simulink model "MPC_MEKF"  (R2024b)
settings: Solver=ode4  StartTime=0.0  StopTime=tsim  FixedStep=baseRate  RelTol=1e-6  AbsTol=1e-6
values from neighbouring files (symbols this model uses):
  D = zeros(3)    [MPC_Configuration.m]
  FOV = 120    [CV_Configuration.m]
  Gamma1_el = 0.12    [Run_Initializer.m]
  Gamma1_sh = 0.005    [Run_Initializer.m]
  Gamma1_wr = 0.025    [Run_Initializer.m]
  Gamma2_el = 5    [Run_Initializer.m]
  Gamma2_sh = 5    [Run_Initializer.m]
  Gamma2_wr = 5    [Run_Initializer.m]
  Gamma3_el = 10    [Run_Initializer.m]
  Gamma3_sh = 40    [Run_Initializer.m]
  Gamma3_wr = 40    [Run_Initializer.m]
  Gamma4_el = 0.039    [Run_Initializer.m]
  Gamma4_sh = 0.015    [Run_Initializer.m]
  Gamma4_wr = 0.029    [Run_Initializer.m]
  Gamma5_el = 800    [Run_Initializer.m]
  Gamma5_sh = 800    [Run_Initializer.m]
  Gamma5_wr = 800    [Run_Initializer.m]
  Gamma6_el = 0.000001    (= 1e-06)    [Run_Initializer.m]
  Gamma6_sh = 0.005    [Run_Initializer.m]
  Gamma6_wr = 0.02    [Run_Initializer.m]
  Kd_elarm = 0.8    [Run_Initializer.m]
  Kd_sharm = 1.0    (= 1)    [Run_Initializer.m]
  Kd_wrarm = 0.6    [Run_Initializer.m]
  kfObs = kfChaser    [PS_Filter_Config.m]
  kfTarget = kfChaser    [PS_Filter_Config.m]
  Kp_elarm = 1.2    [Run_Initializer.m]
  Kp_sharm = 1.5    [Run_Initializer.m]
  Kp_wrarm = 1.0    (= 1)    [Run_Initializer.m]
  M = 1    [MPC_Configuration.m]
  mpcIC = zeros((3*N + 6*N),1)    [MPC_Configuration.m]
  N = 15    [MPC_Configuration.m]    (also in PlotRawCV.m = length(time))
  PWMFreq = 5    [Run_Initializer.m]
  spotKFP0 = zeros(6,6,3)    [PS_Filter_Config.m]
  spotKFx0 = zeros(6,3)    [PS_Filter_Config.m]
  std = 1.5    [CV_Configuration.m]
  Tz_lim_elarm = .1    (= 0.1)    [Run_Initializer.m]
  Tz_lim_sharm = .1    (= 0.1)    [Run_Initializer.m]
  Tz_lim_wrarm = .1    (= 0.1)    [Run_Initializer.m]
  umax = T_max.*[1; 1; (0.3/2)]    [MPC_Configuration.m]
undefined symbols (not defined in the file or in its folder): a1, a2, a3, b0, b1, b2, b3, baseRate, dataRate, DiscIntNeverNeededParam, drop_states_ARM, drop_states_BLACK, drop_states_BLUE, drop_states_RED, F_black_X_nominal, F_black_Y_nominal, F_blue_X_nominal, F_blue_Y_nominal, F_red_X_nominal, F_red_Y_nominal, F_thrusters_BLACK, F_thrusters_BLUE, F_thrusters_RED, home_states_BLACK, home_states_BLUE, home_states_RED, IBLACK, IBLUE, IDIST, IEE, init_states_BLACK, init_states_BLUE, init_states_RED, IPROX, IRED, K_BLACK, K_BLUE, K_RED, Kd_tb, Kd_tblue, Kd_tr, Kd_xb, Kd_xblue, Kd_xr, Kd_yb, Kd_yblue, Kd_yr, kfChaser, Kp_tb, Kp_tblue, Kp_tr, Kp_xb, Kp_xblue, Kp_xr, Kp_yb, Kp_yblue, Kp_yr, mBLACK, mBLUE, mDIST ... (+23)
libraries: simulink x30, nvidiaSharedBlocks x13, MainLibrary x5, dspinverses x3, nvidiaIMUSensorslib x1
(part 2 of 8)

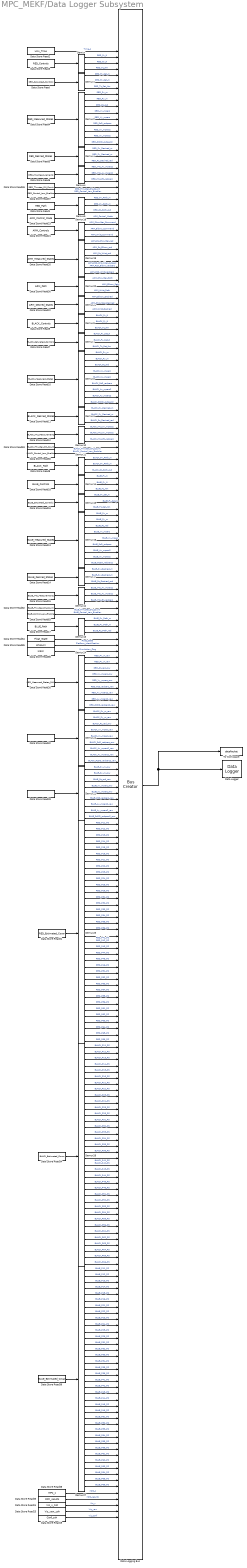
== system MPC_MEKF/Data Logger Subsystem ==
  Data Logger : MainLibrary/Data Logger  SystemSampleTime=-1  VariantActivationTime=update diagram  AllowFlexibleInterface=on  Latency=0  AutoFrameSizeCalculation=off
      settings: SourceProductName=SPOT Custom Library
  Data Logging Bus : BusCreator  Inputs=238
  Data Store Read : DataStoreRead  DataStoreName=RED_Saturated_Controls  IndexOptions=Index vector (dialog)  Indices=1  OutputSizes=1
  Data Store Read1 : DataStoreRead  DataStoreName=RED_Path  IndexOptions=Index vector (dialog)  Indices=1  OutputSizes=1
  Data Store Read10 : DataStoreRead  DataStoreName=BLACK_Measured_States  IndexOptions=Index vector (dialog)  Indices=1  OutputSizes=1
  Data Store Read11 : DataStoreRead  DataStoreName=BLACK_Desired_States  IndexOptions=Index vector (dialog)  Indices=1  OutputSizes=1
  Data Store Read12 : DataStoreRead  DataStoreName=BLACK_IMU_Measurements  IndexOptions=Index vector (dialog)  Indices=1  OutputSizes=1
  Data Store Read13 : DataStoreRead  DataStoreName=BLUE_Measured_States  IndexOptions=Index vector (dialog)  Indices=1  OutputSizes=1
  Data Store Read14 : DataStoreRead  DataStoreName=BLUE_Desired_States  IndexOptions=Index vector (dialog)  Indices=1  OutputSizes=1
  Data Store Read15 : DataStoreRead  DataStoreName=BLUE_IMU_Measurements  IndexOptions=Index vector (dialog)  Indices=1  OutputSizes=1
  Data Store Read16 : DataStoreRead  DataStoreName=BLUE_Saturated_Controls  IndexOptions=Index vector (dialog)  Indices=1  OutputSizes=1
  Data Store Read17 : DataStoreRead  DataStoreName=BLUE_Path  IndexOptions=Index vector (dialog)  Indices=1  OutputSizes=1
  Data Store Read18 : DataStoreRead  DataStoreName=BLUE_Controls  IndexOptions=Index vector (dialog)  Indices=1  OutputSizes=1
  Data Store Read19 : DataStoreRead  DataStoreName=Conf_zoh  IndexOptions=Index vector (dialog)  Indices=1  OutputSizes=1
  Data Store Read2 : DataStoreRead  DataStoreName=Univ_Time  IndexOptions=Index vector (dialog)  Indices=1  OutputSizes=1
  Data Store Read20 : DataStoreRead  DataStoreName=ARM_Measured_States  IndexOptions=Index vector (dialog)  Indices=1  OutputSizes=1
  Data Store Read21 : DataStoreRead  DataStoreName=ARM_Controls  IndexOptions=Index vector (dialog)  Indices=1  OutputSizes=1
  Data Store Read22 : DataStoreRead  DataStoreName=ARM_Desired_States  IndexOptions=Index vector (dialog)  Indices=1  OutputSizes=1
  Data Store Read23 : DataStoreRead  DataStoreName=ARM_Control_Mode  IndexOptions=Index vector (dialog)  Indices=1  OutputSizes=1
  Data Store Read24 : DataStoreRead  DataStoreName=Vis_x_zoh  IndexOptions=Index vector (dialog)  Indices=1  OutputSizes=1
  Data Store Read25 : DataStoreRead  DataStoreName=Vis_yaw_zoh  IndexOptions=Index vector (dialog)  Indices=1  OutputSizes=1
  Data Store Read26 : DataStoreRead  DataStoreName=RED_Measured_States_RAW  IndexOptions=Index vector (dialog)  Indices=1  OutputSizes=1
  Data Store Read28 : DataStoreRead  DataStoreName=BLUE_Measured_States_RAW  IndexOptions=Index vector (dialog)  Indices=1  OutputSizes=1
  Data Store Read3 : DataStoreRead  DataStoreName=RED_Controls  IndexOptions=Index vector (dialog)  Indices=1  OutputSizes=1
  Data Store Read30 : DataStoreRead  DataStoreName=ARM_Path  IndexOptions=Index vector (dialog)  Indices=1  OutputSizes=1
  Data Store Read31 : DataStoreRead  DataStoreName=RED_Estimated_Covar  IndexOptions=Index vector (dialog)  Indices=1  OutputSizes=1
  Data Store Read32 : DataStoreRead  DataStoreName=BLACK_Measured_States_RAW  IndexOptions=Index vector (dialog)  Indices=1  OutputSizes=1
  Data Store Read34 : DataStoreRead  DataStoreName=BLACK_Estimated_Covar  IndexOptions=Index vector (dialog)  Indices=1  OutputSizes=1
  Data Store Read35 : DataStoreRead  DataStoreName=MPC_results  IndexOptions=Index vector (dialog)  Indices=1  OutputSizes=1
  Data Store Read36 : DataStoreRead  DataStoreName=RED_Thruster_ON_Count  IndexOptions=Index vector (dialog)  Indices=1  OutputSizes=1
  Data Store Read37 : DataStoreRead  DataStoreName=RED_Control_Law_Enabler  IndexOptions=Index vector (dialog)  Indices=1  OutputSizes=1
  Data Store Read38 : DataStoreRead  DataStoreName=MPC_z  IndexOptions=Index vector (dialog)  Indices=1  OutputSizes=1
  Data Store Read39 : DataStoreRead  DataStoreName=BLUE_Estimated_Covar  IndexOptions=Index vector (dialog)  Indices=1  OutputSizes=1
  Data Store Read4 : DataStoreRead  DataStoreName=RED_Measured_States  IndexOptions=Index vector (dialog)  Indices=1  OutputSizes=1
  Data Store Read5 : DataStoreRead  DataStoreName=RED_Desired_States  IndexOptions=Index vector (dialog)  Indices=1  OutputSizes=1
  Data Store Read59 : DataStoreRead  DataStoreName=BLACK_Thruster_ON_Count  IndexOptions=Index vector (dialog)  Indices=1  OutputSizes=1
  Data Store Read6 : DataStoreRead  DataStoreName=RED_IMU_Measurements  IndexOptions=Index vector (dialog)  Indices=1  OutputSizes=1
  Data Store Read60 : DataStoreRead  DataStoreName=BLACK_Control_Law_Enabler  IndexOptions=Index vector (dialog)  Indices=1  OutputSizes=1
  Data Store Read7 : DataStoreRead  DataStoreName=BLACK_Saturated_Controls  IndexOptions=Index vector (dialog)  Indices=1  OutputSizes=1
  Data Store Read8 : DataStoreRead  DataStoreName=BLACK_Path  IndexOptions=Index vector (dialog)  Indices=1  OutputSizes=1
  Data Store Read82 : DataStoreRead  DataStoreName=BLUE_Thruster_ON_Count  IndexOptions=Index vector (dialog)  Indices=1  OutputSizes=1
  Data Store Read83 : DataStoreRead  DataStoreName=BLUE_Control_Law_Enabler  IndexOptions=Index vector (dialog)  Indices=1  OutputSizes=1
  Data Store Read84 : DataStoreRead  DataStoreName=Float_State  IndexOptions=Index vector (dialog)  Indices=1  OutputSizes=1
  Data Store Read85 : DataStoreRead  DataStoreName=WhoAmI  IndexOptions=Index vector (dialog)  Indices=1  OutputSizes=1
  Data Store Read86 : DataStoreRead  DataStoreName=isSim  IndexOptions=Index vector (dialog)  Indices=1  OutputSizes=1
  Data Store Read9 : DataStoreRead  DataStoreName=BLACK_Controls  IndexOptions=Index vector (dialog)  Indices=1  OutputSizes=1
  Demux{,1,3..7,9..15,17..18,20..21} (18 alike) : Demux  Outputs=3
  Demux{2,8,16,22..24} (6 alike) : Demux  Outputs=9
  Demux19 : Demux  Outputs=6
  Demux25 : Demux  Outputs=36
  Demux26 : Demux  Outputs=36
  Demux27 : Demux  Outputs=36
  To Workspace : ToWorkspace  VariableName=dataPacket  SaveFormat=Timeseries  SampleTime=-1
      settings: Save2DSignal=2-D array (concatenate along first dimension)
  wires:
  Data Logging Bus/1 -> To Workspace/1, Data Logger/1
  Demux6/1 -> Data Logging Bus/44  "BLACK_Fx_N"
  Demux6/2 -> Data Logging Bus/45  "BLACK_Fy_N"
  Demux6/3 -> Data Logging Bus/46  "BLACK_Tz_Nm"
  Demux7/1 -> Data Logging Bus/47  "BLACK_Fx_Sat_N"
  Demux7/2 -> Data Logging Bus/48  "BLACK_Fy_Sat_N"
  Demux7/3 -> Data Logging Bus/49  "BLACK_Tz_Sat_Nm"
  Demux8/1 -> Data Logging Bus/50  "BLACK_Px_m"
  Demux8/2 -> Data Logging Bus/51  "BLACK_Py_m"
  Demux8/3 -> Data Logging Bus/52  "BLACK_Rz_rad"
  Demux8/4 -> Data Logging Bus/53  "BLACK_Vx_mpers"
  Demux8/5 -> Data Logging Bus/54  "BLACK_Vy_mpers"
  Demux8/6 -> Data Logging Bus/55  "BLACK_RzD_radpers"
  Demux8/7 -> Data Logging Bus/56  "BLACK_Ax_mpers2"
  Demux8/8 -> Data Logging Bus/57  "BLACK_Ay_mpers2"
  Demux8/9 -> Data Logging Bus/58  "BLACK_RzDD_radpers2"
  Demux9/1 -> Data Logging Bus/59  "BLACK_Px_Desired_m"
  Demux9/2 -> Data Logging Bus/60  "BLACK_Py_Desired_m"
  Demux9/3 -> Data Logging Bus/61  "BLACK_Rz_Desired_rad"
  Demux10/1 -> Data Logging Bus/62  "BLACK_IMU_Ax_mpers2"
  Demux10/2 -> Data Logging Bus/63  "BLACK_IMU_Ay_mpers2"
  Demux10/3 -> Data Logging Bus/64  "BLACK_IMU_Gz_radpers"
  Demux11/1 -> Data Logging Bus/67  "BLACK_Px_Path_m"
  Demux11/2 -> Data Logging Bus/68  "BLACK_Py_Path_m"
  Demux11/3 -> Data Logging Bus/69  "BLACK_Rz_Path_rad"
  Demux14/1 -> Data Logging Bus/70  "BLUE_Fx_N"
  Demux14/2 -> Data Logging Bus/71  "BLUE_Fy_N"
  Demux14/3 -> Data Logging Bus/72  "BLUE_Tz_Nm"
  Demux15/1 -> Data Logging Bus/73  "BLUE_Fx_Sat_N"
  Demux15/2 -> Data Logging Bus/74  "BLUE_Fy_Sat_N"
  Demux15/3 -> Data Logging Bus/75  "BLUE_Tz_Sat_Nm"
  Demux16/1 -> Data Logging Bus/76  "BLUE_Px_m"
  Demux16/2 -> Data Logging Bus/77  "BLUE_Py_m"
  Demux16/3 -> Data Logging Bus/78  "BLUE_Rz_rad"
  Demux16/4 -> Data Logging Bus/79  "BLUE_Vx_mpers"
  Demux16/5 -> Data Logging Bus/80  "BLUE_Vy_mpers"
  Demux16/6 -> Data Logging Bus/81  "BLUE_RzD_radpers"
  Demux16/7 -> Data Logging Bus/82  "BLUE_Ax_mpers2"
  Demux16/8 -> Data Logging Bus/83  "BLUE_Ay_mpers2"
  Demux16/9 -> Data Logging Bus/84  "BLUE_RzDD_radpers2"
  Demux17/1 -> Data Logging Bus/85  "BLUE_Px_Desired_m"
  Demux17/2 -> Data Logging Bus/86  "BLUE_Py_Desired_m"
  Demux17/3 -> Data Logging Bus/87  "BLUE_Rz_Desired_rad"
  Demux12/1 -> Data Logging Bus/88  "BLUE_IMU_Ax_mpers2"
  Demux12/2 -> Data Logging Bus/89  "BLUE_IMU_Ay_mpers2"
  Demux12/3 -> Data Logging Bus/90  "BLUE_IMU_Gz_radpers"
  Data Store Read82/1 -> Data Logging Bus/91  "BLUE_Thruster_ON_Count"
  Data Store Read83/1 -> Data Logging Bus/92  "BLUE_Control_Law_Enabler"
  Demux13/1 -> Data Logging Bus/93  "BLUE_Px_Path_m"
  Demux13/2 -> Data Logging Bus/94  "BLUE_Py_Path_m"
  Demux13/3 -> Data Logging Bus/95  "BLUE_Rz_Path_rad"
  Data Store Read86/1 -> Data Logging Bus/98  "Simulation_Flag"
  Demux21/3 -> Data Logging Bus/43  "ARM_Wrist_Desired"
  Demux21/2 -> Data Logging Bus/42  "ARM_Shoulder_Desired"
  Demux21/1 -> Data Logging Bus/41  "ARM_Elbow_Desired"
  Demux20/3 -> Data Logging Bus/40  "ARM_Wrist_Path"
  Demux20/2 -> Data Logging Bus/39  "ARM_Elbow_Path"
  Data Store Read23/1 -> Data Logging Bus/28  "ARM_Control_Mode"
  Demux18/1 -> Data Logging Bus/29  "ARM_Shoulder_Command"
  Demux18/2 -> Data Logging Bus/30  "ARM_Elbow_Command"
  Demux18/3 -> Data Logging Bus/31  "ARM_Wrist_Command"
  Demux19/1 -> Data Logging Bus/32  "ARM_Rz_Shoulder_rad"
  Demux19/2 -> Data Logging Bus/33  "ARM_Rz_Elbow_rad"
  Demux19/3 -> Data Logging Bus/34  "ARM_Rz_Wrist_rad"
  Demux19/4 -> Data Logging Bus/35  "ARM_RzD_Shoulder_radpers"
  Demux19/5 -> Data Logging Bus/36  "ARM_RzD_Elbow_radpers"
  Demux19/6 -> Data Logging Bus/37  "ARM_RzD_Wrist_radpers"
  Demux20/1 -> Data Logging Bus/38  "ARM_Shoulder_Path"
  Data Store Read2/1 -> Data Logging Bus/1  "Time_s"
  Demux/1 -> Data Logging Bus/2  "RED_Fx_N"
  Demux/2 -> Data Logging Bus/3  "RED_Fy_N"
  Demux/3 -> Data Logging Bus/4  "RED_Tz_Nm"
  Demux1/1 -> Data Logging Bus/5  "RED_Fx_Sat_N"
  Demux1/2 -> Data Logging Bus/6  "RED_Fy_Sat_N"
  Demux1/3 -> Data Logging Bus/7  "RED_Tz_Sat_Nm"
  Demux2/1 -> Data Logging Bus/8  "RED_Px_m"
  Demux2/2 -> Data Logging Bus/9  "RED_Py_m"
  Demux2/3 -> Data Logging Bus/10  "RED_Rz_rad"
  Demux2/4 -> Data Logging Bus/11  "RED_Vx_mpers"
  Demux2/5 -> Data Logging Bus/12  "RED_Vy_mpers"
  Demux2/6 -> Data Logging Bus/13  "RED_RzD_radpers"
  Demux2/7 -> Data Logging Bus/14  "RED_Ax_mpers2"
  Demux2/8 -> Data Logging Bus/15  "RED_Ay_mpers2"
  Demux2/9 -> Data Logging Bus/16  "RED_RzDD_radpers2"
  Demux3/1 -> Data Logging Bus/17  "RED_Px_Desired_m"
  Demux3/2 -> Data Logging Bus/18  "RED_Py_Desired_m"
  Demux3/3 -> Data Logging Bus/19  "RED_Rz_Desired_rad"
  Demux4/1 -> Data Logging Bus/20  "RED_IMU_Ax_mpers2"
  Demux4/2 -> Data Logging Bus/21  "RED_IMU_Ay_mpers2"
  Demux4/3 -> Data Logging Bus/22  "RED_IMU_Gz_radpers"
  Data Store Read36/1 -> Data Logging Bus/23  "RED_Thruster_ON_Count"
  Data Store Read37/1 -> Data Logging Bus/24  "RED_Control_Law_Enabler"
  Demux5/1 -> Data Logging Bus/25  "RED_Px_Path_m"
  Demux5/2 -> Data Logging Bus/26  "RED_Py_Path_m"
  Demux5/3 -> Data Logging Bus/27  "RED_Rz_Path_rad"
  Data Store Read/1 -> Demux1/1
  Data Store Read3/1 -> Demux/1
  Data Store Read4/1 -> Demux2/1
  Data Store Read5/1 -> Demux3/1
  Data Store Read6/1 -> Demux4/1
  Data Store Read1/1 -> Demux5/1
  Data Store Read12/1 -> Demux10/1
  Data Store Read8/1 -> Demux11/1
  Data Store Read10/1 -> Demux8/1
  Data Store Read7/1 -> Demux7/1
  Data Store Read9/1 -> Demux6/1
  Data Store Read11/1 -> Demux9/1
  Data Store Read18/1 -> Demux14/1
  Data Store Read17/1 -> Demux13/1
  Data Store Read13/1 -> Demux16/1
  Data Store Read16/1 -> Demux15/1
  Data Store Read15/1 -> Demux12/1
  Data Store Read14/1 -> Demux17/1
  Data Store Read21/1 -> Demux18/1
  Data Store Read20/1 -> Demux19/1
  Data Store Read30/1 -> Demux20/1
  Data Store Read22/1 -> Demux21/1
  Data Store Read85/1 -> Data Logging Bus/97  "Platform_Identification"
  Data Store Read59/1 -> Data Logging Bus/65  "BLACK_Thruster_ON_Count"
  Data Store Read60/1 -> Data Logging Bus/66  "BLACK_Control_Law_Enabler"
  Data Store Read84/1 -> Data Logging Bus/96  "Float_State"
  Demux24/1 -> Data Logging Bus/99  "RED_Px_m_raw"
  Demux22/9 -> Data Logging Bus/125  "BLUE_RzDD_radpers2_raw"
  Data Store Read26/1 -> Demux24/1
  Demux24/2 -> Data Logging Bus/100  "RED_Py_m_raw"
  Demux24/3 -> Data Logging Bus/101  "RED_Rz_rad_raw"
  Demux24/4 -> Data Logging Bus/102  "RED_Vx_mpers_raw"
  Demux24/5 -> Data Logging Bus/103  "RED_Vy_mpers_raw"
  Demux24/6 -> Data Logging Bus/104  "RED_RzD_radpers_raw"
  Demux24/7 -> Data Logging Bus/105  "RED_Ax_mpers2_raw"
  Demux24/8 -> Data Logging Bus/106  "RED_Ay_mpers2_raw"
  Demux24/9 -> Data Logging Bus/107  "RED_RzDD_radpers2_raw"
  Demux23/1 -> Data Logging Bus/108  "BLACK_Px_m_raw"
  Demux23/2 -> Data Logging Bus/109  "BLACK_Py_m_raw"
  Demux23/3 -> Data Logging Bus/110  "BLACK_Rz_rad_raw"
  Demux23/4 -> Data Logging Bus/111  "BLACK_Vx_mpers_raw"
  Demux23/5 -> Data Logging Bus/112  "BLACK_Vy_mpers_raw"
  Demux23/6 -> Data Logging Bus/113  "BLACK_RzD_radpers_raw"
  Demux23/7 -> Data Logging Bus/114  "BLACK_Ax_mpers2_raw"
  Demux23/8 -> Data Logging Bus/115  "BLACK_Ay_mpers2_raw"
  Demux23/9 -> Data Logging Bus/116  "BLACK_RzDD_radpers2_raw"
  Data Store Read32/1 -> Demux23/1
  Demux22/1 -> Data Logging Bus/117  "BLUE_Px_m_raw"
  Demux22/2 -> Data Logging Bus/118  "BLUE_Py_m_raw"
  Demux22/3 -> Data Logging Bus/119  "BLUE_Rz_rad_raw"
  Demux22/4 -> Data Logging Bus/120  "BLUE_Vx_mpers_raw"
  Demux22/5 -> Data Logging Bus/121  "BLUE_Vy_mpers_raw"
  Demux22/6 -> Data Logging Bus/122  "BLUE_RzD_radpers_raw"
  Demux22/7 -> Data Logging Bus/123  "BLUE_Ax_mpers2_raw"
  Demux22/8 -> Data Logging Bus/124  "BLUE_Ay_mpers2_raw"
  Data Store Read28/1 -> Demux22/1
  Demux25/1 -> Data Logging Bus/126  "RED_P11_PS"
  Demux25/2 -> Data Logging Bus/127  "RED_P12_PS"
  Demux25/3 -> Data Logging Bus/128  "RED_P13_PS"
  Demux25/4 -> Data Logging Bus/129  "RED_P14_PS"
  Demux25/5 -> Data Logging Bus/130  "RED_P15_PS"
  Demux25/6 -> Data Logging Bus/131  "RED_P16_PS"
  Demux25/7 -> Data Logging Bus/132  "RED_P21_PS"
  Demux25/8 -> Data Logging Bus/133  "RED_P22_PS"
  Demux25/9 -> Data Logging Bus/134  "RED_P23_PS"
  Demux25/10 -> Data Logging Bus/135  "RED_P24_PS"
  Demux25/11 -> Data Logging Bus/136  "RED_P25_PS"
  Demux25/12 -> Data Logging Bus/137  "RED_P26_PS"
  Demux25/13 -> Data Logging Bus/138  "RED_P31_PS"
  Demux25/14 -> Data Logging Bus/139  "RED_P32_PS"
  Demux25/15 -> Data Logging Bus/140  "RED_P33_PS"
  Demux25/16 -> Data Logging Bus/141  "RED_P34_PS"
  Demux25/17 -> Data Logging Bus/142  "RED_P35_PS"
  Demux25/18 -> Data Logging Bus/143  "RED_P36_PS"
  Demux25/19 -> Data Logging Bus/144  "RED_P41_PS"
  Demux25/20 -> Data Logging Bus/145  "RED_P42_PS"
  Demux25/21 -> Data Logging Bus/146  "RED_P43_PS"
  Demux25/22 -> Data Logging Bus/147  "RED_P44_PS"
  Demux25/23 -> Data Logging Bus/148  "RED_P45_PS"
  Demux25/24 -> Data Logging Bus/149  "RED_P46_PS"
  Demux25/25 -> Data Logging Bus/150  "RED_P51_PS"
  Demux25/26 -> Data Logging Bus/151  "RED_P52_PS"
  Demux25/27 -> Data Logging Bus/152  "RED_P53_PS"
  Demux25/28 -> Data Logging Bus/153  "RED_P54_PS"
  Demux25/29 -> Data Logging Bus/154  "RED_P55_PS"
  Demux25/30 -> Data Logging Bus/155  "RED_P56_PS"
  Demux25/31 -> Data Logging Bus/156  "RED_P61_PS"
  Demux25/32 -> Data Logging Bus/157  "RED_P62_PS"
  Demux25/33 -> Data Logging Bus/158  "RED_P63_PS"
  Demux25/34 -> Data Logging Bus/159  "RED_P64_PS"
  Demux25/35 -> Data Logging Bus/160  "RED_P65_PS"
  Demux25/36 -> Data Logging Bus/161  "RED_P66_PS"
  Data Store Read31/1 -> Demux25/1
  Demux26/1 -> Data Logging Bus/162  "BLACK_P11_PS"
  Demux26/2 -> Data Logging Bus/163  "BLACK_P12_PS"
  Demux26/3 -> Data Logging Bus/164  "BLACK_P13_PS"
  Demux26/4 -> Data Logging Bus/165  "BLACK_P14_PS"
  Demux26/5 -> Data Logging Bus/166  "BLACK_P15_PS"
  Demux26/6 -> Data Logging Bus/167  "BLACK_P16_PS"
  Demux26/7 -> Data Logging Bus/168  "BLACK_P21_PS"
  Demux26/8 -> Data Logging Bus/169  "BLACK_P22_PS"
  Demux26/9 -> Data Logging Bus/170  "BLACK_P23_PS"
  Demux26/10 -> Data Logging Bus/171  "BLACK_P24_PS"
  Demux26/11 -> Data Logging Bus/172  "BLACK_P25_PS"
  Demux26/12 -> Data Logging Bus/173  "BLACK_P26_PS"
  Demux26/13 -> Data Logging Bus/174  "BLACK_P31_PS"
  Demux26/14 -> Data Logging Bus/175  "BLACK_P32_PS"
  Demux26/15 -> Data Logging Bus/176  "BLACK_P33_PS"
  Demux26/16 -> Data Logging Bus/177  "BLACK_P34_PS"
  Demux26/17 -> Data Logging Bus/178  "BLACK_P35_PS"
  Demux26/18 -> Data Logging Bus/179  "BLACK_P36_PS"
  Demux26/19 -> Data Logging Bus/180  "BLACK_P41_PS"
  Demux26/20 -> Data Logging Bus/181  "BLACK_P42_PS"
  Demux26/21 -> Data Logging Bus/182  "BLACK_P43_PS"
  Demux26/22 -> Data Logging Bus/183  "BLACK_P44_PS"
  Demux26/23 -> Data Logging Bus/184  "BLACK_P45_PS"
  Demux26/24 -> Data Logging Bus/185  "BLACK_P46_PS"
  Demux26/25 -> Data Logging Bus/186  "BLACK_P51_PS"
  Demux26/26 -> Data Logging Bus/187  "BLACK_P52_PS"
  Demux26/27 -> Data Logging Bus/188  "BLACK_P53_PS"
  Demux26/28 -> Data Logging Bus/189  "BLACK_P54_PS"
  Demux26/29 -> Data Logging Bus/190  "BLACK_P55_PS"
  Demux26/30 -> Data Logging Bus/191  "BLACK_P56_PS"
  Demux26/31 -> Data Logging Bus/192  "BLACK_P61_PS"
  Demux26/32 -> Data Logging Bus/193  "BLACK_P62_PS"
  Demux26/33 -> Data Logging Bus/194  "BLACK_P63_PS"
  Demux26/34 -> Data Logging Bus/195  "BLACK_P64_PS"
  Demux26/35 -> Data Logging Bus/196  "BLACK_P65_PS"
  Demux26/36 -> Data Logging Bus/197  "BLACK_P66_PS"
  Data Store Read34/1 -> Demux26/1
  Demux27/1 -> Data Logging Bus/198  "BLUE_P11_PS"
  Demux27/2 -> Data Logging Bus/199  "BLUE_P12_PS"
  Demux27/3 -> Data Logging Bus/200  "BLUE_P13_PS"
  Demux27/4 -> Data Logging Bus/201  "BLUE_P14_PS"
  Demux27/5 -> Data Logging Bus/202  "BLUE_P15_PS"
  Demux27/6 -> Data Logging Bus/203  "BLUE_P16_PS"
  Demux27/7 -> Data Logging Bus/204  "BLUE_P21_PS"
  Demux27/8 -> Data Logging Bus/205  "BLUE_P22_PS"
  Demux27/9 -> Data Logging Bus/206  "BLUE_P23_PS"
  Demux27/10 -> Data Logging Bus/207  "BLUE_P24_PS"
  Demux27/11 -> Data Logging Bus/208  "BLUE_P25_PS"
  Demux27/12 -> Data Logging Bus/209  "BLUE_P26_PS"
  Demux27/13 -> Data Logging Bus/210  "BLUE_P31_PS"
  Demux27/14 -> Data Logging Bus/211  "BLUE_P32_PS"
  Demux27/15 -> Data Logging Bus/212  "BLUE_P33_PS"
  Demux27/16 -> Data Logging Bus/213  "BLUE_P34_PS"
  Demux27/17 -> Data Logging Bus/214  "BLUE_P35_PS"
  Demux27/18 -> Data Logging Bus/215  "BLUE_P36_PS"
  Demux27/19 -> Data Logging Bus/216  "BLUE_P41_PS"
  Demux27/20 -> Data Logging Bus/217  "BLUE_P42_PS"
  Demux27/21 -> Data Logging Bus/218  "BLUE_P43_PS"
  Demux27/22 -> Data Logging Bus/219  "BLUE_P44_PS"
  Demux27/23 -> Data Logging Bus/220  "BLUE_P45_PS"
  Demux27/24 -> Data Logging Bus/221  "BLUE_P46_PS"
  Demux27/25 -> Data Logging Bus/222  "BLUE_P51_PS"
  Demux27/26 -> Data Logging Bus/223  "BLUE_P52_PS"
  Demux27/27 -> Data Logging Bus/224  "BLUE_P53_PS"
  Demux27/28 -> Data Logging Bus/225  "BLUE_P54_PS"
  Demux27/29 -> Data Logging Bus/226  "BLUE_P55_PS"
  Demux27/30 -> Data Logging Bus/227  "BLUE_P56_PS"
  Demux27/31 -> Data Logging Bus/228  "BLUE_P61_PS"
  Demux27/32 -> Data Logging Bus/229  "BLUE_P62_PS"
  Demux27/33 -> Data Logging Bus/230  "BLUE_P63_PS"
  Demux27/34 -> Data Logging Bus/231  "BLUE_P64_PS"
  Demux27/35 -> Data Logging Bus/232  "BLUE_P65_PS"
  Demux27/36 -> Data Logging Bus/233  "BLUE_P66_PS"
  Data Store Read39/1 -> Demux27/1
  Data Store Read38/1 -> Data Logging Bus/234  "MPC_z"
  Data Store Read35/1 -> Data Logging Bus/235  "MPC_results"
  Data Store Read24/1 -> Data Logging Bus/236  "Vis_x"
  Data Store Read25/1 -> Data Logging Bus/237  "Vis_yaw"
  Data Store Read19/1 -> Data Logging Bus/238  "Vis_conf"

== system MPC_MEKF/Debugger ==
  Change BLACK Behavior : Subsystem  TreatAsAtomicUnit=on
  Change BLUE Behavior : Subsystem  TreatAsAtomicUnit=on
  Change RED Behavior : Subsystem  TreatAsAtomicUnit=on
  Data Store Read : DataStoreRead  DataStoreName=WhoAmI  IndexOptions=Index vector (dialog)  Indices=1  OutputSizes=1
  Data Store Read1 : DataStoreRead  DataStoreName=isSim  IndexOptions=Index vector (dialog)  Indices=1  OutputSizes=1
  This IF block determines whether or not to run the BLACK sim/exp : If  NumInputs=2  IfExpression=u1 == 2 & u2 == 0  ShowElse=off
  This IF block determines whether or not to run the BLUE sim/exp : If  NumInputs=2  IfExpression=u1 == 3 & u2 == 0  ShowElse=off
  "This IF block determines whether or not to run the RED sim/exp " : If  NumInputs=2  IfExpression=u1 == 1 & u2 == 0  ShowElse=off
  wires:
  This IF block determines whether or not to run the BLUE sim/exp/1 -> Change BLUE Behavior/Action
  Data Store Read1/1 -> This IF block determines whether or not to run the BLACK sim/exp/2, This IF block determines whether or not to run the BLUE sim/exp/2, "This IF block determines whether or not to run the RED sim/exp "/2
  "This IF block determines whether or not to run the RED sim/exp "/1 -> Change RED Behavior/Action
  Data Store Read/1 -> This IF block determines whether or not to run the BLUE sim/exp/1, This IF block determines whether or not to run the BLACK sim/exp/1, "This IF block determines whether or not to run the RED sim/exp "/1
  This IF block determines whether or not to run the BLACK sim/exp/1 -> Change BLACK Behavior/Action

== system MPC_MEKF/Float Code ==
  note: In this subsection, the "if" statements are used to determine two things: 1) whether or not a simulation is begin performed,
      | then 2) if an experiment is being performed, then which platform is the diagram compiled on. The "IdentifyPlatform" variable
      | is obtained from a text file location on each platform; each text file contains a unique identifier for each platform.
  Data Store Read : DataStoreRead  DataStoreName=isSim  IndexOptions=Index vector (dialog)  Indices=1  OutputSizes=1
  Enable Pucks : Subsystem  TreatAsAtomicUnit=on
  This IF block determines whether or not to run the exp code : If  IfExpression=u1 == 0  ShowElse=off
  wires:
  Data Store Read/1 -> This IF block determines whether or not to run the exp code/1
  This IF block determines whether or not to run the exp code/1 -> Enable Pucks/Action

== system MPC_MEKF/Gyro.//Accel. Code ==
  Data Store Read1 : DataStoreRead  DataStoreName=isSim  IndexOptions=Index vector (dialog)  Indices=1  OutputSizes=1
  Log Gyro/Accel : Subsystem  TreatAsAtomicUnit=on
  This IF block determines whether or not to run the exp code : If  IfExpression=u1 == 0  ShowElse=off
  wires:
  This IF block determines whether or not to run the exp code/1 -> Log Gyro/Accel/Action
  Data Store Read1/1 -> This IF block determines whether or not to run the exp code/1

== system MPC_MEKF/MPC ==
  Data Store Read : DataStoreRead  DataStoreName=RED_Measured_States  IndexOptions=Index vector (dialog)  Indices=1  OutputSizes=1
  Data Store Read1 : DataStoreRead  DataStoreName=BLACK_Measured_States  IndexOptions=Index vector (dialog)  Indices=1  OutputSizes=1
  Data Store Read2 : DataStoreRead  DataStoreName=BLUE_Measured_States  IndexOptions=Index vector (dialog)  Indices=1  OutputSizes=1
  Data Store Read3 : DataStoreRead  DataStoreName=RED_Estimated_Covar  IndexOptions=Index vector (dialog)  Indices=1  OutputSizes=1
  Data Store Read4 : DataStoreRead  DataStoreName=BLACK_Estimated_Covar  IndexOptions=Index vector (dialog)  Indices=1  OutputSizes=1
  Data Store Read5 : DataStoreRead  DataStoreName=BLUE_Estimated_Covar  IndexOptions=Index vector (dialog)  Indices=1  OutputSizes=1
  Data Store Write : DataStoreWrite  DataStoreName=MPC_results  IndexOptions=Index vector (dialog)  Indices=1  OutputSizes=1
  Data Store Write1 : DataStoreWrite  DataStoreName=MPC_z  IndexOptions=Index vector (dialog)  Indices=1  OutputSizes=1
  Data Store Write2 : DataStoreWrite  DataStoreName=MPC_u  IndexOptions=Index vector (dialog)  Indices=1  OutputSizes=1
  MPC : MATLAB Function  TreatAsAtomicUnit=on
  Memory : Memory  InitialCondition=mpcIC  InheritSampleTime=on
  Reshape4 : Reshape
  wires:
  Data Store Read5/1 -> MPC/7(P_Obs)
  MPC/3(results) -> Reshape4/1
  Data Store Read1/1 -> MPC/4(x_targ)
  Data Store Read4/1 -> MPC/5(P_targ)
  Data Store Read/1 -> MPC/2(x_chase)
  Reshape4/1 -> Data Store Write/1
  MPC/1(z) -> Memory/1, Data Store Write1/1
  Data Store Read3/1 -> MPC/3(P_chase)
  Memory/1 -> MPC/1(z_prev)
  Data Store Read2/1 -> MPC/6(x_Obs)
  MPC/2(u) -> Data Store Write2/1  "force"

== system MPC_MEKF/Manipulator Encoder Data ==
  note: This if statement checks if a simulation is being performed. If not, it also checks that this code is being run on the RED platform. If it is, then the arm encoders are used to collect the joint angles. NOTE, the encoder data is collected very slowly, about 0.5 Hz. When the diagram is running faster then this collection rate, previous values of the encoder are held constant.
  Change ARM Behavior : Subsystem  TreatAsAtomicUnit=on
  Data Store Read1 : DataStoreRead  DataStoreName=WhoAmI  IndexOptions=Index vector (dialog)  Indices=1  OutputSizes=1
  Data Store Read2 : DataStoreRead  DataStoreName=isSim  IndexOptions=Index vector (dialog)  Indices=1  OutputSizes=1
  "This IF block determines whether or not to run the RED sim/exp " : If  NumInputs=2  IfExpression=u1 == 1 & u2 == 0  ShowElse=off
  wires:
  Data Store Read2/1 -> "This IF block determines whether or not to run the RED sim/exp "/2
  "This IF block determines whether or not to run the RED sim/exp "/1 -> Change ARM Behavior/Action
  Data Store Read1/1 -> "This IF block determines whether or not to run the RED sim/exp "/1

== system MPC_MEKF/PhaseSpace Camera Code ==
  note: In this subsection, the "if" statement is used to determine if this is a simulation or not. If it is not a simulation, then code is run to receive PhaseSpace camera data via UDP. The PhaseSpace code is currently a standalone executable that should not need to be modified by most users. The code sends all data for all platforms to each platform near simultaneously. If this is a simulation, then no data is required, but a continuous clock is created.
  Data Store Read2 : DataStoreRead  DataStoreName=isSim  IndexOptions=Index vector (dialog)  Indices=1  OutputSizes=1
  "If performing an experiment, grab the PhaseSpace data. Otherwise, use a clock to set time in SIM." : If  IfExpression=u1 == 0  ElseIfExpressions=u1 == 1  ShowElse=off
  Initialize Universal Time (Simulation) : Subsystem  TreatAsAtomicUnit=on
  Use Hardware to Obtain States : Subsystem  TreatAsAtomicUnit=on
  wires:
  Data Store Read2/1 -> "If performing an experiment, grab the PhaseSpace data. Otherwise, use a clock to set time in SIM."/1
  "If performing an experiment, grab the PhaseSpace data. Otherwise, use a clock to set time in SIM."/2 -> Initialize Universal Time (Simulation)/Action
  "If performing an experiment, grab the PhaseSpace data. Otherwise, use a clock to set time in SIM."/1 -> Use Hardware to Obtain States/Action

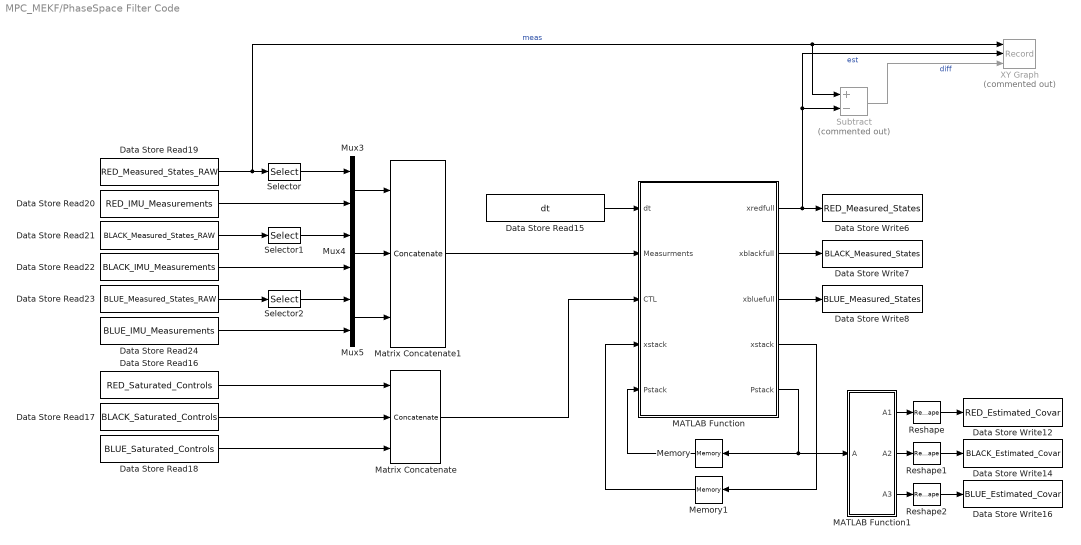
== system MPC_MEKF/PhaseSpace Filter Code ==
  Data Store Read15 : DataStoreRead  DataStoreName=dt  IndexOptions=Index vector (dialog)  Indices=1  OutputSizes=1
  Data Store Read16 : DataStoreRead  DataStoreName=RED_Saturated_Controls  IndexOptions=Index vector (dialog)  Indices=1  OutputSizes=1
  Data Store Read17 : DataStoreRead  DataStoreName=BLACK_Saturated_Controls  IndexOptions=Index vector (dialog)  Indices=1  OutputSizes=1
  Data Store Read18 : DataStoreRead  DataStoreName=BLUE_Saturated_Controls  IndexOptions=Index vector (dialog)  Indices=1  OutputSizes=1
  Data Store Read19 : DataStoreRead  DataStoreName=RED_Measured_States_RAW  IndexOptions=Index vector (dialog)  Indices=1  OutputSizes=1
  Data Store Read20 : DataStoreRead  DataStoreName=RED_IMU_Measurements  IndexOptions=Index vector (dialog)  Indices=1  OutputSizes=1
  Data Store Read21 : DataStoreRead  DataStoreName=BLACK_Measured_States_RAW  IndexOptions=Index vector (dialog)  Indices=1  OutputSizes=1
  Data Store Read22 : DataStoreRead  DataStoreName=BLACK_IMU_Measurements  IndexOptions=Index vector (dialog)  Indices=1  OutputSizes=1
  Data Store Read23 : DataStoreRead  DataStoreName=BLUE_Measured_States_RAW  IndexOptions=Index vector (dialog)  Indices=1  OutputSizes=1
  Data Store Read24 : DataStoreRead  DataStoreName=BLUE_IMU_Measurements  IndexOptions=Index vector (dialog)  Indices=1  OutputSizes=1
  Data Store Write12 : DataStoreWrite  DataStoreName=RED_Estimated_Covar  IndexOptions=Index vector (dialog)  Indices=1  OutputSizes=1
  Data Store Write14 : DataStoreWrite  DataStoreName=BLACK_Estimated_Covar  IndexOptions=Index vector (dialog)  Indices=1  OutputSizes=1
  Data Store Write16 : DataStoreWrite  DataStoreName=BLUE_Estimated_Covar  IndexOptions=Index vector (dialog)  Indices=1  OutputSizes=1
  Data Store Write6 : DataStoreWrite  DataStoreName=RED_Measured_States  IndexOptions=Index vector (dialog)  Indices=1  OutputSizes=1
  Data Store Write7 : DataStoreWrite  DataStoreName=BLACK_Measured_States  IndexOptions=Index vector (dialog)  Indices=1  OutputSizes=1
  Data Store Write8 : DataStoreWrite  DataStoreName=BLUE_Measured_States  IndexOptions=Index vector (dialog)  Indices=1  OutputSizes=1
  MATLAB Function : MATLAB Function  TreatAsAtomicUnit=on
  MATLAB Function1 : MATLAB Function  TreatAsAtomicUnit=on
  Matrix Concatenate : Concatenate  NumInputs=3  Mode=Multidimensional array  ConcatenateDimension=2
  Matrix Concatenate1 : Concatenate  NumInputs=3  Mode=Multidimensional array  ConcatenateDimension=2
  Memory : Memory  InitialCondition=spotKFP0
  Memory1 : Memory  InitialCondition=spotKFx0
  Mux3 : Mux  Inputs=2
  Mux4 : Mux  Inputs=2
  Mux5 : Mux  Inputs=2
  Reshape : Reshape
  Reshape1 : Reshape
  Reshape2 : Reshape
  Selector : Selector  InputPortWidth=9  IndexOptions=Index vector (dialog)  Indices=[1:3]  OutputSizes=1
  Selector1 : Selector  InputPortWidth=9  IndexOptions=Index vector (dialog)  Indices=[1:3]  OutputSizes=1
  Selector2 : Selector  InputPortWidth=9  IndexOptions=Index vector (dialog)  Indices=[1:3]  OutputSizes=1
  Subtract : Sum  Commented=on  Inputs=+-
  XY Graph : Record  Commented=on  FileSettingsInternal="{\"entries\":[{\"content\":{\"excelSettings\":{\"content\":{},\"type\":\"Streamout.ExcelSettings\"}},\"type\":\"Streamout.FileSettingStorage\",\"uuid\":\"\"}],\"packageUris\":[\"http:\\/\\/schema.mathworks.com\\/mf0\\/streamout_blocks\\/R2020a\"],\"version\":\"1.0\"}"  Layout=[1 1]  SignalsInternal="{\"entries\":[{\"content\":{},\"type\":\"RecordBlkView.InputSignals\",\"uuid\":\"\"}],\"packageUris\":[\"http:\\/\\/schema.mathworks.com\\/mf0\\/streamout_blocks\\/R2020a\"],\"version\":\"1.0\"}"  VisualizationBindings="{\"sparklinesplugin\":{\"info\":[{\"bindingParametersList\":[],\"subplotID\":1}]}}"  CompatibilityTag=XY
  wires:
  Data Store Read15/1 -> MATLAB Function/1(dt)
  Data Store Read16/1 -> Matrix Concatenate/1
  Data Store Read17/1 -> Matrix Concatenate/2
  Data Store Read18/1 -> Matrix Concatenate/3
  Data Store Read21/1 -> Selector1/1
  Data Store Read22/1 -> Mux4/2
  Data Store Read19/1 -> Subtract/1, XY Graph/1, Selector/1  "meas"
  Data Store Read20/1 -> Mux3/2
  Data Store Read23/1 -> Selector2/1
  Data Store Read24/1 -> Mux5/2
  Mux5/1 -> Matrix Concatenate1/3
  Mux4/1 -> Matrix Concatenate1/2
  Mux3/1 -> Matrix Concatenate1/1
  Matrix Concatenate1/1 -> MATLAB Function/2(Measurments)
  Matrix Concatenate/1 -> MATLAB Function/3(CTL)
  Selector/1 -> Mux3/1
  Selector1/1 -> Mux4/1
  Selector2/1 -> Mux5/1
  Memory/1 -> MATLAB Function/5("Pstack ")
  MATLAB Function/5(Pstack) -> Memory/1, MATLAB Function1/1(A)
  Memory1/1 -> MATLAB Function/4("xstack ")
  MATLAB Function/4(xstack) -> Memory1/1
  MATLAB Function/1(xredfull) -> Subtract/2, XY Graph/2, Data Store Write6/1  "est"
  MATLAB Function/2(xblackfull) -> Data Store Write7/1
  MATLAB Function/3(xbluefull) -> Data Store Write8/1
  MATLAB Function1/2(A2) -> Reshape1/1
  MATLAB Function1/3(A3) -> Reshape2/1
  MATLAB Function1/1(A1) -> Reshape/1
  Reshape/1 -> Data Store Write12/1
  Reshape1/1 -> Data Store Write14/1
  Reshape2/1 -> Data Store Write16/1
  Subtract/1 -> XY Graph/3  "diff"

== system MPC_MEKF/Platform Identification ==
  Data Store Read1 : DataStoreRead  DataStoreName=isSim  IndexOptions=Index vector (dialog)  Indices=1  OutputSizes=1
  "If 'simMode' set to '1', then this is a simulation and the dynamics will be simulated. Otherwise, this is an experiment, and the simulation will not be run." : If  IfExpression=u1 == 0  ShowElse=off
  Subsystem : Subsystem
  wires:
  "If 'simMode' set to '1', then this is a simulation and the dynamics will be simulated. Otherwise, this is an experiment, and the simulation will not be run."/1 -> Subsystem/Action
  Data Store Read1/1 -> "If 'simMode' set to '1', then this is a simulation and the dynamics will be simulated. Otherwise, this is an experiment, and the simulation will not be run."/1

== system MPC_MEKF/Receive Data  ==
  Cast To Double4 : DataTypeConversion  OutDataTypeStr=double  SaturateOnIntegerOverflow=off  RndMeth=Floor
  Data Store Read : DataStoreRead  DataStoreName=RED_True_States  IndexOptions=Index vector (dialog)  Indices=1  OutputSizes=1
  Data Store Read1 : DataStoreRead  DataStoreName=BLACK_True_States  IndexOptions=Index vector (dialog)  Indices=1  OutputSizes=1
  Data Store Read2 : DataStoreRead  DataStoreName=BLUE_True_States  IndexOptions=Index vector (dialog)  Indices=1  OutputSizes=1
  Data Store Write1 : DataStoreWrite  DataStoreName=Conf  IndexOptions=Index vector (dialog)  Indices=1  OutputSizes=1
  Data Store Write13 : DataStoreWrite  DataStoreName=Vis_dq_zoh  IndexOptions=Index vector (dialog)  Indices=1  OutputSizes=1
  Data Store Write14 : DataStoreWrite  DataStoreName=Vis_q_zoh  IndexOptions=Index vector (dialog)  Indices=1  OutputSizes=1
  Data Store Write15 : DataStoreWrite  DataStoreName=Vis_R_zoh  IndexOptions=Index vector (dialog)  Indices=1  OutputSizes=1
  Data Store Write18 : DataStoreWrite  DataStoreName=Vis_x_zoh  IndexOptions=Index vector (dialog)  Indices=1  OutputSizes=1
  Data Store Write19 : DataStoreWrite  DataStoreName=Vis_dq  IndexOptions=Index vector (dialog)  Indices=1  OutputSizes=1
  Data Store Write2 : DataStoreWrite  DataStoreName=Conf_zoh  IndexOptions=Index vector (dialog)  Indices=1  OutputSizes=1
  Data Store Write20 : DataStoreWrite  DataStoreName=Vis_q  IndexOptions=Index vector (dialog)  Indices=1  OutputSizes=1
  Data Store Write21 : DataStoreWrite  DataStoreName=Vis_R  IndexOptions=Index vector (dialog)  Indices=1  OutputSizes=1
  Data Store Write22 : DataStoreWrite  DataStoreName=Vis_yaw_zoh  IndexOptions=Index vector (dialog)  Indices=1  OutputSizes=1
  Data Store Write23 : DataStoreWrite  DataStoreName=Vis_yaw  IndexOptions=Index vector (dialog)  Indices=1  OutputSizes=1
  Data Store Write24 : DataStoreWrite  DataStoreName=Vis_x  IndexOptions=Index vector (dialog)  Indices=1  OutputSizes=1
  MATLAB Function2 : MATLAB Function  TreatAsAtomicUnit=on
  UDP Receive1 : nvidiaSharedBlocks/UDP Receive  localURL='0.0.0.0'  localPort=30172  remoteURL='0.0.0.0'  remotePort=-1  recvBufferSize=8192  signalDatatype=single  dims=4  isVarSize=off  showBlockingTime=off  blockingTime=0  sampletime=baseRate  blockPlatform=NVIDIA
  noise generator : Subsystem
  wires:
  UDP Receive1/2 -> MATLAB Function2/2(flag)
  Cast To Double4/1 -> MATLAB Function2/1(UDP)
  MATLAB Function2/8(visZOH_yaw) -> Data Store Write22/1
  MATLAB Function2/9(visZOH_conf) -> Data Store Write2/1
  MATLAB Function2/7(visZOH_x) -> Data Store Write18/1
  MATLAB Function2/3(vis_conf) -> Data Store Write1/1
  MATLAB Function2/10(visZOH_R) -> Data Store Write15/1
  Data Store Read2/1 -> MATLAB Function2/5(xblue)
  noise generator/1(noise) -> MATLAB Function2/6(noise)
  Data Store Read1/1 -> MATLAB Function2/4(xblack)
  Data Store Read/1 -> MATLAB Function2/3(xRed)
  MATLAB Function2/12(visZOH_dq) -> Data Store Write13/1
  MATLAB Function2/5(vis_dq) -> Data Store Write19/1
  MATLAB Function2/1(vis_x) -> Data Store Write24/1
  MATLAB Function2/11(visZOH_q) -> Data Store Write14/1
  MATLAB Function2/2(vis_yaw) -> Data Store Write23/1
  UDP Receive1/1 -> Cast To Double4/1
  MATLAB Function2/6(vis_q) -> Data Store Write20/1
  MATLAB Function2/4(vis_R) -> Data Store Write21/1

== system MPC_MEKF/Robotic Arm Code ==
  note: In this subsection, the "if" statements are used to determine two things: 1) whether or not a simulation is begin performed,
      | then 2) if an experiment is being performed, then which platform is the diagram compiled on. The "IdentifyPlatform" variable
      | is obtained using a custom C++ function which gets the computer name for each platform. NOTE that the arm code only runs on RED.
  Change ARM Behavior : Subsystem  TreatAsAtomicUnit=on
  Data Store Read : DataStoreRead  DataStoreName=WhoAmI  IndexOptions=Index vector (dialog)  Indices=1  OutputSizes=1
  Data Store Read1 : DataStoreRead  DataStoreName=isSim  IndexOptions=Index vector (dialog)  Indices=1  OutputSizes=1
  "This IF block determines whether or not to run the RED sim/exp " : If  NumInputs=2  IfExpression=u1 == 1 & u2 == 0  ShowElse=off
  wires:
  "This IF block determines whether or not to run the RED sim/exp "/1 -> Change ARM Behavior/Action
  Data Store Read1/1 -> "This IF block determines whether or not to run the RED sim/exp "/2
  Data Store Read/1 -> "This IF block determines whether or not to run the RED sim/exp "/1

== system MPC_MEKF/Send Data to Orin ==
  Data Store Read1 : DataStoreRead  DataStoreName=isSim  IndexOptions=Index vector (dialog)  Indices=1  OutputSizes=1
  "If 'simMode' set to '1', then this is a simulation and the dynamics will be simulated. Otherwise, this is an experiment, and the simulation will not be run." : If  IfExpression=u1 == 0  ShowElse=off
  Subsystem : Subsystem
  wires:
  "If 'simMode' set to '1', then this is a simulation and the dynamics will be simulated. Otherwise, this is an experiment, and the simulation will not be run."/1 -> Subsystem/Action
  Data Store Read1/1 -> "If 'simMode' set to '1', then this is a simulation and the dynamics will be simulated. Otherwise, this is an experiment, and the simulation will not be run."/1

== system MPC_MEKF/Simulate Plant Dynamics ==
  Action Port : ActionPort  ActionPortLabel=if(u1 == 1)
  BLACK Dynamics : Subsystem
  BLUE Dynamics : Subsystem
  RED and ARM Dynamics : Subsystem

== system MPC_MEKF/Simulation Status ==
  Constant : Constant  Value=simMode  SampleTime=-1
  Data Store Write : DataStoreWrite  DataStoreName=isSim  IndexOptions=Index vector (dialog)  Indices=1  OutputSizes=1
  wires:
  Constant/1 -> Data Store Write/1

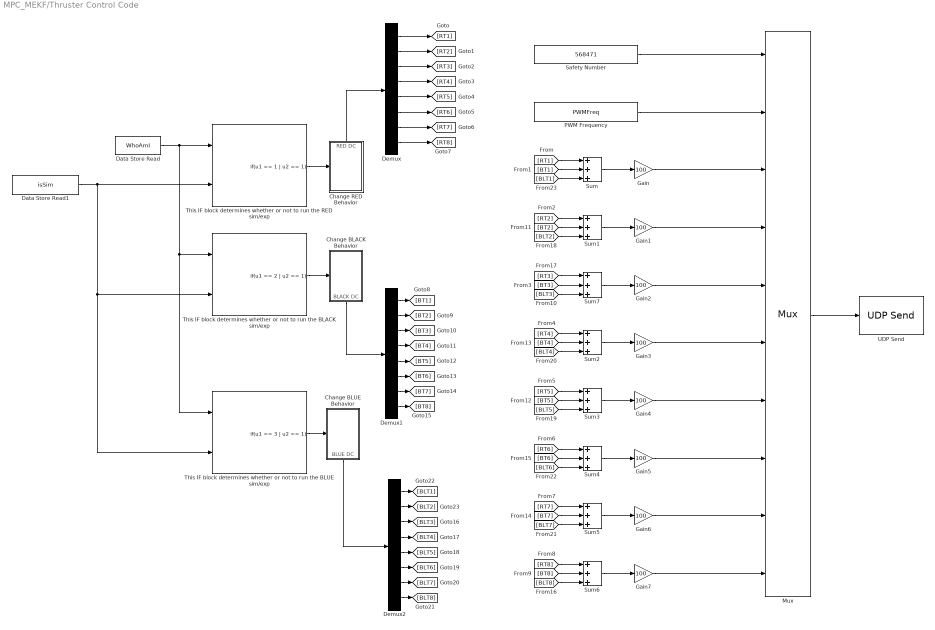
== system MPC_MEKF/Thruster Control Code ==
  Change BLACK Behavior : Subsystem  TreatAsAtomicUnit=on
  Change BLUE Behavior : Subsystem  TreatAsAtomicUnit=on
  Change RED Behavior : Subsystem  TreatAsAtomicUnit=on
  Data Store Read : DataStoreRead  DataStoreName=WhoAmI  IndexOptions=Index vector (dialog)  Indices=1  OutputSizes=1
  Data Store Read1 : DataStoreRead  DataStoreName=isSim  IndexOptions=Index vector (dialog)  Indices=1  OutputSizes=1
  Demux : Demux  Outputs=8
  Demux1 : Demux  Outputs=8
  Demux2 : Demux  Outputs=8
  Gain{,1..7} (8 alike) : Gain  Gain=100
  Mux : Mux  Inputs=10
  PWM Frequency : Constant  Value=PWMFreq
  Safety Number : Constant  Value=568471
  Sum{,1..7} (8 alike) : Sum  Inputs=+++
  This IF block determines whether or not to run the BLACK sim/exp : If  NumInputs=2  IfExpression=u1 == 2 | u2 == 1  ShowElse=off
  This IF block determines whether or not to run the BLUE sim/exp : If  NumInputs=2  IfExpression=u1 == 3 | u2 == 1  ShowElse=off
  "This IF block determines whether or not to run the RED sim/exp " : If  NumInputs=2  IfExpression=u1 == 1 | u2 == 1  ShowElse=off
  UDP Send : nvidiaSharedBlocks/UDP Send  remoteURL='127.0.0.1'  remotePort=48291  localURL='0.0.0.0'  localPortSource=Automatically determine  localPort=-1  sampletime=-1  blockPlatform=NVIDIA  separateLengthPort=0
      settings: LibrarySourceBlock=nvidiaNetworklib/UDP Send
  wires:
  Data Store Read1/1 -> This IF block determines whether or not to run the BLACK sim/exp/2, This IF block determines whether or not to run the BLUE sim/exp/2, "This IF block determines whether or not to run the RED sim/exp "/2
  "This IF block determines whether or not to run the RED sim/exp "/1 -> Change RED Behavior/Action
  This IF block determines whether or not to run the BLACK sim/exp/1 -> Change BLACK Behavior/Action
  Change RED Behavior/1(RED DC) -> Demux/1
  Demux/1 -> [RT1]
  Demux/2 -> [RT2]
  Demux/3 -> [RT3]
  Demux/4 -> [RT4]
  Demux/5 -> [RT5]
  Demux/6 -> [RT6]
  Demux/7 -> [RT7]
  Demux/8 -> [RT8]
  Demux1/5 -> [BT5]
  Demux1/4 -> [BT4]
  Demux1/1 -> [BT1]
  Demux1/8 -> [BT8]
  Demux1/2 -> [BT2]
  Demux1/7 -> [BT7]
  Demux1/6 -> [BT6]
  Demux1/3 -> [BT3]
  Change BLACK Behavior/1(BLACK DC) -> Demux1/1
  Data Store Read/1 -> This IF block determines whether or not to run the BLUE sim/exp/1, This IF block determines whether or not to run the BLACK sim/exp/1, "This IF block determines whether or not to run the RED sim/exp "/1
  This IF block determines whether or not to run the BLUE sim/exp/1 -> Change BLUE Behavior/Action
  Demux2/5 -> [BLT5]
  Demux2/8 -> [BLT8]
  Demux2/7 -> [BLT7]
  Demux2/2 -> [BLT2]
  Change BLUE Behavior/1(BLUE DC) -> Demux2/1
  Demux2/1 -> [BLT1]
  Demux2/4 -> [BLT4]
  Demux2/3 -> [BLT3]
  Demux2/6 -> [BLT6]
  [BT5] -> Sum3/2
  [RT4] -> Sum2/1
  Sum3/1 -> Gain4/1
  [RT2] -> Sum1/1
  [BLT4] -> Sum2/3
  [BT3] -> Sum7/2
  [RT5] -> Sum3/1
  PWM Frequency/1 -> Mux/2
  Gain3/1 -> Mux/6
  [BT8] -> Sum6/2
  Gain7/1 -> Mux/10
  Sum6/1 -> Gain7/1
  Sum7/1 -> Gain2/1
  [BT4] -> Sum2/2
  [RT7] -> Sum5/1
  [BLT3] -> Sum7/3
  Gain1/1 -> Mux/4
  Gain/1 -> Mux/3
  [BLT5] -> Sum3/3
  Sum1/1 -> Gain1/1
  Sum2/1 -> Gain3/1
  Gain4/1 -> Mux/7
  [BLT6] -> Sum4/3
  [BT6] -> Sum4/2
  [BT2] -> Sum1/2
  [BLT2] -> Sum1/3
  [RT1] -> Sum/1
  Sum/1 -> Gain/1
  [BT7] -> Sum5/2
  Gain6/1 -> Mux/9
  [BLT7] -> Sum5/3
  [RT8] -> Sum6/1
  [RT6] -> Sum4/1
  Mux/1 -> UDP Send/1
  [BLT8] -> Sum6/3
  [BT1] -> Sum/2
  Sum5/1 -> Gain6/1
  Gain5/1 -> Mux/8
  Sum4/1 -> Gain5/1
  [BLT1] -> Sum/3
  Safety Number/1 -> Mux/1
  [RT3] -> Sum7/1
  Gain2/1 -> Mux/5

== system MPC_MEKF/dt ==
  Data Store Read6 : DataStoreRead  DataStoreName=Univ_Time  IndexOptions=Index vector (dialog)  Indices=1  OutputSizes=1
  Delay : Delay  DelayLength=1  InputProcessing=Columns as channels (frame based)
  Subtract : Sum  Inputs=+-
  Out1 : Outport
  wires:
  Delay/1 -> Subtract/2
  Subtract/1 -> Out1/1
  Data Store Read6/1 -> Subtract/1, Delay/1

== system MPC_MEKF/1 - Experiment Logic/Phase #0: Synchronization ==
  note: Setting the RED thrusters to OFF.
  note: Setting the PUCKS for ALL to OFF.
  note: DISABLE ARM Path Planning.
  note: Setting the BLACK thrusters to OFF.
  note: Setting the BLUE thrusters to OFF.
  note: DISABLE RED Path Planning.
  note: DISABLE BLACK Path Planning.
  note: DISABLE BLUE Path Planning.
  note: DISABLE ARM Control.
  Action Port : ActionPort  ActionPortLabel=if(u1 < u2)
  Constant{1..8} (8 alike) : Constant  Value=0
  Data Store Write : DataStoreWrite  DataStoreName=RED_Control_Law_Enabler  IndexOptions=Index vector (dialog)  Indices=1  OutputSizes=1
  Data Store Write1 : DataStoreWrite  DataStoreName=RED_Logger  IndexOptions=Index vector (dialog)  Indices=1  OutputSizes=1
  Data Store Write2 : DataStoreWrite  DataStoreName=BLACK_Control_Law_Enabler  IndexOptions=Index vector (dialog)  Indices=1  OutputSizes=1
  Data Store Write3 : DataStoreWrite  DataStoreName=BLUE_Control_Law_Enabler  IndexOptions=Index vector (dialog)  Indices=1  OutputSizes=1
  Data Store Write4 : DataStoreWrite  DataStoreName=Float_State  IndexOptions=Index vector (dialog)  Indices=1  OutputSizes=1
  Data Store Write5 : DataStoreWrite  DataStoreName=BLUE_Path_Planner_Selection  IndexOptions=Index vector (dialog)  Indices=1  OutputSizes=1
  Data Store Write6 : DataStoreWrite  DataStoreName=BLACK_Path_Planner_Selection  IndexOptions=Index vector (dialog)  Indices=1  OutputSizes=1
  Data Store Write7 : DataStoreWrite  DataStoreName=RED_Path_Planner_Selection  IndexOptions=Index vector (dialog)  Indices=1  OutputSizes=1
  Data Store Write8 : DataStoreWrite  DataStoreName=ARM_Path_Planner_Selection  IndexOptions=Index vector (dialog)  Indices=1  OutputSizes=1
  Data Store Write9 : DataStoreWrite  DataStoreName=ARM_Control_Law_Enabler  IndexOptions=Index vector (dialog)  Indices=1  OutputSizes=1
  Puck State : Constant  Value=0
  String Constant : StringConstant  String="\"Chaser: Running Phase 0\""
  wires:
  Constant4/1 -> Data Store Write8/1
  Puck State/1 -> Data Store Write4/1
  Constant5/1 -> Data Store Write/1
  Constant1/1 -> Data Store Write2/1
  Constant2/1 -> Data Store Write3/1
  Constant3/1 -> Data Store Write7/1
  Constant6/1 -> Data Store Write6/1
  Constant7/1 -> Data Store Write5/1
  Constant8/1 -> Data Store Write9/1
  String Constant/1 -> Data Store Write1/1
